simulink model "unidade3TestarBomba"  (R2015b)
settings: Solver=ode1  StartTime=0.0  StopTime=inf  FixedStep=0.002  RelTol=1e-3
PostLoadFcn:
  | qc_set_target_type(getConfigSet(bdroot, 'QUARC Default Target Configuration'));
undefined symbols (not defined in the file or in its folder): HIL
libraries: quarc_library x3
settings Model: SimulationMode=external  ExtModeTrigDuration=30000  Creator=MLevis  LastModifiedBy=UFRN
settings SolverCC: PositivePriorityOrder=on
settings DataIOCC: SaveFormat=Array  SignalLoggingSaveFormat=ModelDataLogs
settings OptimizationCC: ExpressionDepthLimit=2147483647  InitFltsAndDblsToZero=on
settings DebuggingCC: SaveWithParameterizedLinksMsg=none  UnderspecifiedInitializationDetection=Classic  MergeDetectMultiDrivingBlocksExec=none  SolverPrmCheckMsg=warning  MultiTaskDSMMsg=warning  MultiTaskCondExecSysMsg=none  FcnCallInpInsideContextMsg=UseLocalSettings  StateNameClashWarn=warning
settings HardwareCC: ProdBitPerPointer=32  ProdLargestAtomicFloat=None  ProdIntDivRoundTo=Undefined  ProdEndianess=Unspecified  ProdWordSize=32  ProdHWDeviceType=32-bit Generic
settings RTWCC: SystemTargetFile=quarc_win64.tlc  TemplateMakefile=quarc_default_tmf  Description=QUARC Win64 Target
settings GRTTargetCC: ParMdlRefBuildCompliant=off  CompOptLevelCompliant=off  GeneratePreprocessorConditionals=Disable all  CombineOutputUpdateFcns=off  MatFileLogging=off  GRTInterface=on  UseToolchainInfoCompliant=off  ExtMode=on  ExtModeMexFile=quarc_comm
settings ConfigComp: CovModelRefEnable=Off

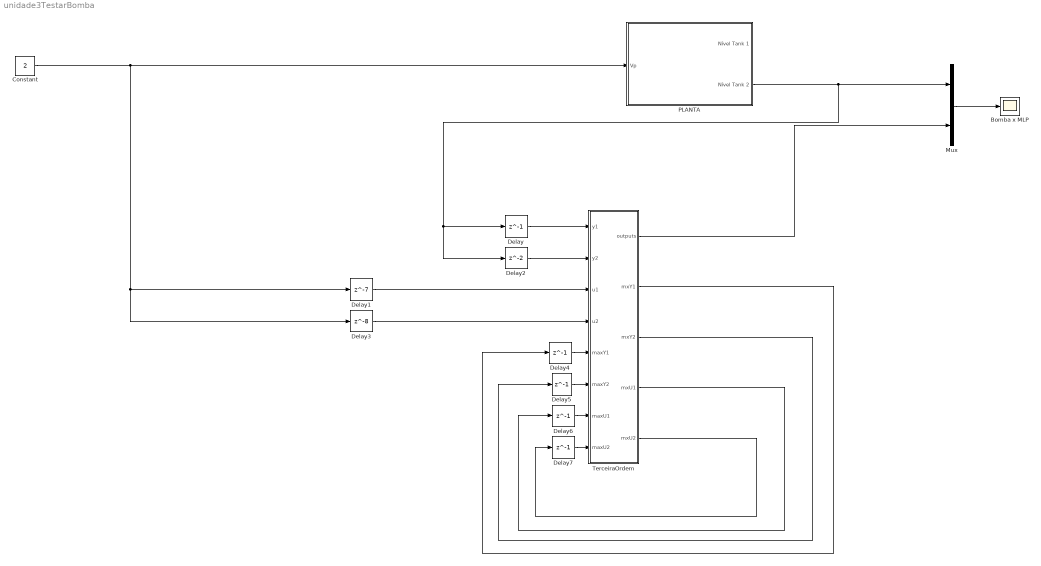
== system unidade3TestarBomba ==
  "Bomba x MLP " : Scope
  Constant : Constant  Value=2
  Delay{,4..7} (5 alike) : Delay  DelayLength=1  InitialCondition=0
  Delay1 : Delay  DelayLength=7  InitialCondition=0
  Delay2 : Delay  InitialCondition=0
  Delay3 : Delay  DelayLength=8  InitialCondition=0
  Mux : Mux  Inputs=2
  PLANTA : Subsystem
  "TerceiraOrdem " : MATLAB Function  TreatAsAtomicUnit=on
  wires:
  Mux/1 -> "Bomba x MLP "/1
  Delay/1 -> "TerceiraOrdem "/1(y1)
  Delay1/1 -> "TerceiraOrdem "/3(u1)
  Delay2/1 -> "TerceiraOrdem "/2(y2)
  Delay3/1 -> "TerceiraOrdem "/4(u2)
  PLANTA/2(Nível Tank 2) -> Delay2/1, Delay/1, Mux/1
  Constant/1 -> Delay3/1, Delay1/1, PLANTA/1(Vp)
  "TerceiraOrdem "/1(outputs) -> Mux/2
  "TerceiraOrdem "/2(mxY1) -> Delay4/1
  "TerceiraOrdem "/3(mxY2) -> Delay5/1
  "TerceiraOrdem "/4(mxU1) -> Delay6/1
  "TerceiraOrdem "/5(mxU2) -> Delay7/1
  Delay4/1 -> "TerceiraOrdem "/5(maxY1)
  Delay5/1 -> "TerceiraOrdem "/6(maxY2)
  Delay6/1 -> "TerceiraOrdem "/7(maxU1)
  Delay7/1 -> "TerceiraOrdem "/8(maxU2)

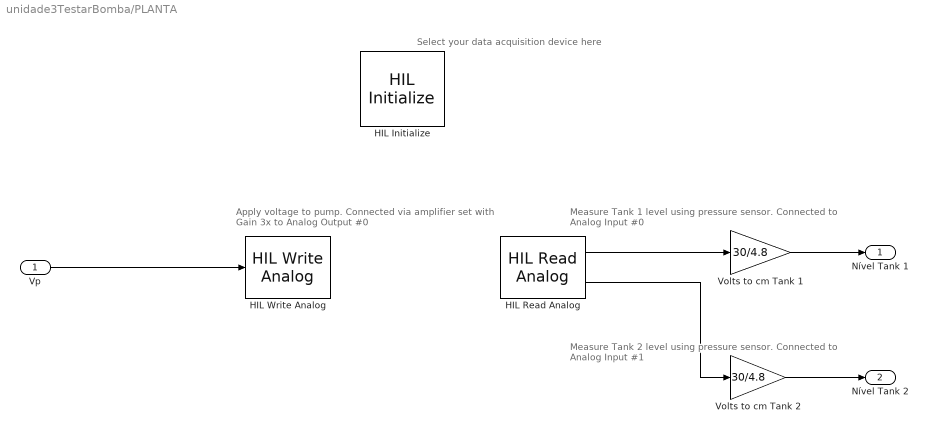
== system unidade3TestarBomba/PLANTA ==
  note: Select your data acquisition device here
  note: Apply voltage to pump.
      | Connected via amplifier set with Gain 3x
      | to  Analog Output #0
  note: Measure Tank 2 level using pressure sensor.
      | Connected to Analog Input #1
  note: Measure Tank 1 level using pressure sensor.
      | Connected to Analog Input #0
  Vp : Inport
  HIL Initialize : quarc_library/Data Acquisition/Generic/Configuration/HIL Initialize  object_name=HIL-1  board_type=q8_usb  board_number=0  board_options=update_rate=normal;decimation=1  exclusive=off  active=off  hardware_clocks=[0:2]  clock_modes=[]  initial_clock_frequencies=[]  set_clock_params_at_start=off  set_clock_params_at_switch_in=off  set_clock_frequencies_at_start=off  set_clock_frequencies_at_switch_in=off  analog_input_channels=[0:7]  analog_input_maximums=10  analog_input_minimums=-10  set_analog_input_params_at_start=on  set_analog_input_params_at_switch_in=off  analog_output_channels=[0:7]  analog_output_maximums=10  analog_output_minimums=-10  initial_analog_outputs=[0]  final_analog_outputs=[0]  watchdog_analog_outputs=0  set_analog_output_params_at_start=on  set_analog_output_params_at_switch_in=off  set_analog_outputs_at_start=on  set_analog_outputs_at_switch_in=off  set_analog_outputs_at_terminate=on  set_analog_outputs_at_switch_out=off  set_analog_outputs_on_watchdog=off  digital_input_channels=[]  digital_output_channels=[]  digital_output_configuration=[]  initial_digital_outputs=[1]  final_digital_outputs=[1]  watchdog_digital_outputs=[1]  set_digital_output_params_at_start=off  set_digital_output_params_at_switch_in=off  set_digital_outputs_at_start=on  set_digital_outputs_at_switch_in=off  set_digital_outputs_at_terminate=on  set_digital_outputs_at_switch_out=off  set_digital_outputs_on_watchdog=off  encoder_channels=[0:7]  quadrature=[4]  encoder_filter_frequency=[]  initial_encoder_counts=[0]  set_encoder_params_at_start=on  set_encoder_params_at_switch_in=off  set_encoder_counts_at_start=on  set_encoder_counts_at_switch_in=off  pwm_channels=[0:7]  pwm_modes=0  pwm_frequency=99.532799999999995e6/4095  pwm_configuration=[0]  pwm_alignment=[0]  pwm_polarity=[1]  pwm_leading_deadband=[0]  pwm_trailing_deadband=[0]  initial_pwm_outputs=[0]  final_pwm_outputs=[0]  watchdog_pwm_outputs=[0]  set_pwm_params_at_start=on  set_pwm_params_at_switch_in=off  set_pwm_outputs_at_start=on  set_pwm_outputs_at_switch_in=off  set_pwm_outputs_at_terminate=on  set_pwm_outputs_at_switch_out=off  set_pwm_outputs_on_watchdog=off  other_output_channels=[]  initial_other_outputs=[]  final_other_outputs=[]  watchdog_other_outputs=[]  set_other_outputs_at_start=off  set_other_outputs_at_switch_in=off  set_other_outputs_at_terminate=off  set_other_outputs_at_switch_out=off  set_other_outputs_on_watchdog=off
  HIL Read Analog : quarc_library/Data Acquisition/Generic/Immediate I//O/HIL Read Analog  object_name=HIL-1  channels=[0:1]  sample_time=qc_get_step_size  active=on  vector_output=off
  HIL Write Analog : quarc_library/Data Acquisition/Generic/Immediate I//O/HIL Write Analog  object_name=HIL-1  channels=0  sample_time=-1  active=off  vector_input=off
  "Volts to cm Tank 1 " : Gain  Gain=30/4.8
  Volts to cm Tank 2 : Gain  Gain=30/4.8
  Nível Tank 1 : Outport
  Nível Tank 2 : Outport  Port=2
  wires:
  HIL Read Analog/1 -> "Volts to cm Tank 1 "/1
  HIL Read Analog/2 -> Volts to cm Tank 2/1
  Vp/1 -> HIL Write Analog/1
  "Volts to cm Tank 1 "/1 -> Nível Tank 1/1
  Volts to cm Tank 2/1 -> Nível Tank 2/1

== matlab function unidade3TestarBomba/TerceiraOrdem  ==
  data: y1 input; y2 input; u1 input; outputs output; u2 input; maxY1 input; maxY2 input; maxU1 input; maxU2 input; mxY1 output; mxY2 output; mxU1 output; mxU2 output
%% Ordem 1, Atraso 1
function [outputs,mxY1,mxY2,mxU1,mxU2] = EvaluateNetworkForSimulink(y1,y2,u1,u2,maxY1,maxY2,maxU1,maxU2)
%nbrOfLayers = length(nce);
PesosIn=[-0.0260    0.2413   -0.9102    0.5803   -0.0162   -0.8738    0.4453   -0.5591   -0.6570    0.1721   -0.8350    0.3728   -0.7091    0.9315   -1.0036   -0.3005   -0.9897    0.0898   -0.9625   -0.1540 0.8795;
    0.0176    0.3014   -0.5584    0.8441   -0.3786    0.9293    0.6061    0.2057   -0.8042   -0.0919    0.1627   -0.9609    1.0180   -0.5312   -0.9459   -0.6517   -0.8978    0.0410   -0.6613    0.7258 -0.5233;
    0.0176    0.8337   -0.7946    0.0613   -0.6051    0.3883   -0.8358   -0.1470   -0.8066    0.1627   -0.6476    0.0870    0.6732   -0.7032    0.3060   -0.1110    0.6957   -0.0411    0.5428   -1.0036 -0.2678;
   -0.0150   -0.5701    0.2674   -0.5106   -0.1702    0.8124    0.2770   -1.0010    0.4380   -0.0459   -0.6791    0.7101    0.7687   -0.2704    0.8221    0.3171    0.9186   -0.3955   -0.9863    0.3217 0.6672;
   -0.0151    0.4670   -0.0873    0.6972   -0.8524   -0.8403    0.9726   -0.2130   -0.8362    0.7906    0.4847    0.0557   -0.7884   -0.4743   -0.3514   -0.6616   -0.0297    0.0677    0.6239    0.4961 -0.7746]
PesosEsc= [0.0962;  0.4341;  -0.2677;   0.3255;  -0.1881;   0.5136;  -0.0558;   0.1161;   -0.2824;    0.0565;   -0.0913;   -0.2677;    0.6539;   -0.3336;   -0.1501;   -0.1768;   -0.0447;    0.0709;    0.0124;   -0.0725;  -0.1937];
PesosOut=1;



maxY1=max(maxY1,y1);
maxY2=max(maxY2,y2);
maxU1=max(maxU1,u1);
maxU2=max(maxU2,u2);

y1=y1./maxY1;
y2=y2./maxY2;
u1=u1./maxU1;
u2=u2./maxU2;

Sample=[y1 y2 u1 u2];
Sample = [ones(length(Sample(:,1)),1) Sample];

NodeIn = Sample;

NodeIn = NodeIn*PesosIn;



NodeIn = FuncaoAtivacao(NodeIn,'LOGSIGMOIDE');

NodeHid=NodeIn;


NodeHid = NodeHid*PesosEsc;

NodeHid = FuncaoAtivacao(NodeHid,'LOGSIGMOIDE');


NodeOut=NodeHid;
NodeOut = NodeOut*PesosOut;

outputs=NodeOut.*max(maxY1,max(maxY2,max(maxU1,maxU2)));

mxY1=maxY1;
mxY2=maxY2;
mxU1=maxU1;
mxU2=maxU2;
end
